simulink model "PFC_ControllerUnit"  (R2021a)
settings: Solver=VariableStepDiscrete  StartTime=0.0  StopTime=20  MaxStep=1/10000  RelTol=1e-3  AbsTol=1e-3
settings Model: PacingRate=1000  Creator=ykamatan  LastModifiedBy=ykamatan
settings SolverCC: AutoScaleAbsTol=off  SolverJacobianMethodControl=SparsePerturbation  DaesscMode=Fast
settings DataIOCC: SaveOutput=off  SaveTime=off
settings DebuggingCC: SymbolicDimsDataTypeCodeGenerationDiagnostic=none  SFMachineParentedDataDiag=warning
settings SFSimCC: CustomCodeUndefinedFunction=UseInterfaceOnly
settings SimscapeCC: SimscapeLogType=all  SimscapeLogSimulationStatistics=on  SimscapeLogDataHistory=10000

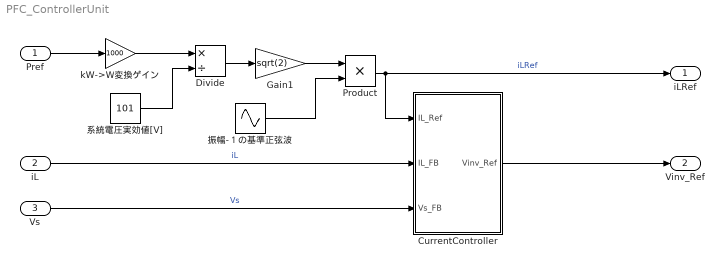
== system PFC_ControllerUnit ==
  Pref : Inport  OutDataTypeStr=double  PortDimensions=1
  iL : Inport  Port=2
  Vs : Inport  Port=3
  CurrentController : Subsystem
  Divide : Product  Inputs=*/
  Gain1 : Gain  Gain=sqrt(2)
  Product : Product
  kW->W変換ゲイン : Gain  Gain=1000
  振幅-１の基準正弦波 : Sin  Amplitude=-1  Frequency=2*pi*60  SampleTime=1/10000
  系統電圧実効値[V] : Constant  Value=101
  iLRef : Outport  OutDataTypeStr=double  PortDimensions=1
  Vinv_Ref : Outport  Port=2  OutDataTypeStr=double  PortDimensions=1
  wires:
  iL/1 -> CurrentController/2(IL_FB)  "iL"
  Pref/1 -> kW->W変換ゲイン/1
  Product/1 -> iLRef/1, CurrentController/1(IL_Ref)  "iLRef"
  振幅-１の基準正弦波/1 -> Product/2
  Gain1/1 -> Product/1
  Vs/1 -> CurrentController/3(Vs_FB)  "Vs"
  CurrentController/1(Vinv_Ref) -> Vinv_Ref/1
  Divide/1 -> Gain1/1
  系統電圧実効値[V]/1 -> Divide/2
  kW->W変換ゲイン/1 -> Divide/1

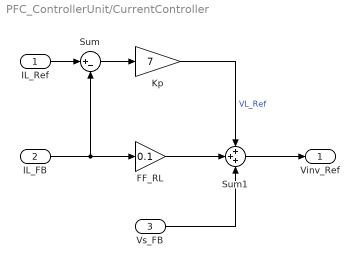
== system PFC_ControllerUnit/CurrentController ==
  IL_Ref : Inport
  IL_FB : Inport  Port=2
  Vs_FB : Inport  Port=3
  FF_RL : Gain  Gain=0.1
  Kp : Gain  Gain=7
  Sum : Sum  Inputs=|+-
  Sum1 : Sum  Inputs=+++
  Vinv_Ref : Outport
  wires:
  FF_RL/1 -> Sum1/2
  Sum1/1 -> Vinv_Ref/1
  Vs_FB/1 -> Sum1/3
  IL_Ref/1 -> Sum/1
  Sum/1 -> Kp/1
  Kp/1 -> Sum1/1  "VL_Ref"
  IL_FB/1 -> Sum/2, FF_RL/1
